simulink model "mdl5"  (R2014a)
settings: Solver=FixedStepDiscrete  SolverMode=SingleTasking  StartTime=TIME(1)  StopTime=TIME(end)  FixedStep=SIMSTEP  RelTol=1e-3
model workspace (MAT data in the model file):
  autoc_mdd_data01 : struct (value not decoded)
values from neighbouring files (symbols this model uses):
  map_mr4_01 = [400 500 600 700 800 900 1000 1100 1200 1300 1400 1500 ... (47 elements, 1x47)]    [scr_simdata_all.mat]
  map_mr4_02 = [0.684 0.622 0.566 0.514 0.468 0.425 0.387 0.352 0.32 0.291 0.264 0.241 ... (47 elements, 1x47)]    [scr_simdata_all.mat]
  map_mr4_03 = [10 12 14 16 18 20 22 24 26 28 30 32 ... (51 elements, 1x51)]    [scr_simdata_all.mat]
  map_mr4_04 = [0.0257 0.0124 0.00595 0.00286 0.00137 0.000662 0.000318 0.000153 7.37e-05 3.54e-05 1.7e-05 8.19e-06 ... (51 elements, 1x51)]    [scr_simdata_all.mat]
  map_mr4_05 = [10 12 14 16 18 20 22 24 26 28 30 32 ... (51 elements, 1x51)]    [scr_simdata_all.mat]
  map_mr4_06 = [0.9647 0.9835 0.9945 0.9994 0.9972 0.9871 0.97 0.9462 0.9163 0.8807 0.8403 0.796 ... (51 elements, 1x51)]    [scr_simdata_all.mat]
  map_mr4_07 = [0 1 2 3 4 5 6 7 8 9 10 11 ... (51 elements, 1x51)]    [scr_simdata_all.mat]
  map_mr4_08 = [0 0.01 0.0214 0.0335 0.0459 0.0587 0.0718 0.085 0.0985 0.112 0.126 0.14 ... (51 elements, 1x51)]    [scr_simdata_all.mat]
  Parameter114 = 126    [scr_simdata_all.mat]
  Parameter115 = 129    [scr_simdata_all.mat]
  Parameter131 = 3    [scr_simdata_all.mat]
  Parameter141 = 0    [scr_simdata_all.mat]
  Parameter143 = 1    [scr_simdata_all.mat]
  Parameter144 = 3    [scr_simdata_all.mat]
  Parameter51 = 0    [scr_simdata_all.mat]
  Parameter52 = 1    [scr_simdata_all.mat]
  Parameter53 = 2    [scr_simdata_all.mat]
  Parameter70 = 30    [scr_simdata_all.mat]
  Parameter71 = 33    [scr_simdata_all.mat]
  Parameter92 = 78    [scr_simdata_all.mat]
  Parameter93 = 81    [scr_simdata_all.mat]
  SIMSTEP = 0.0001024    [scr_simdata_all.mat]
(part 2 of 4)

== system mdl5/SubSystem2611/SubSystem2612/SubSystem2620/SubSystem2621 ==
  note: ***編集禁止***
  element : Inport
  Inside_DSR : DataStoreRead  DataStoreName=DSM320
  Selector : Selector  IndexOptions=Index vector (port)  Indices=[1 3]
  Output : Outport
  wires:
  Selector/1 -> Output/1  "mdl5_SubSystem2611_SubSystem2612_SubSystem2620_SubSystem2621_Selector_1"
  element/1 -> Selector/2
  Inside_DSR/1 -> Selector/1  "mdl5_SubSystem2611_SubSystem2612_SubSystem2620_SubSystem2621_Inside_DSR_1"

== system mdl5/SubSystem2611/SubSystem2612/SubSystem2620/SubSystem2622 ==
  note: ***編集禁止***
  element : Inport
  Inside_DSR : DataStoreRead  DataStoreName=DSM319
  Selector : Selector  IndexOptions=Index vector (port)  Indices=[1 3]
  Output : Outport
  wires:
  Inside_DSR/1 -> Selector/1  "mdl5_SubSystem2611_SubSystem2612_SubSystem2620_SubSystem2622_Inside_DSR_1"
  element/1 -> Selector/2
  Selector/1 -> Output/1  "mdl5_SubSystem2611_SubSystem2612_SubSystem2620_SubSystem2622_Selector_1"

== system mdl5/SubSystem2611/SubSystem2612/SubSystem2620/SubSystem2623 ==
  note: ***編集禁止***
  input : Inport
  element : Inport  Port=2
  Assignment : Assignment  IndexOptions=Index vector (port)  OutputSizes=[1 1]
  Inside_DSR : DataStoreRead  DataStoreName=DSM304
  Inside_DSW : DataStoreWrite  DataStoreName=DSM304
  wires:
  element/1 -> Assignment/3
  input/1 -> Assignment/2
  Inside_DSR/1 -> Assignment/1  "mdl5_SubSystem2611_SubSystem2612_SubSystem2620_SubSystem2623_Inside_DSR_1"
  Assignment/1 -> Inside_DSW/1  "mdl5_SubSystem2611_SubSystem2612_SubSystem2620_SubSystem2623_Assignment_1"

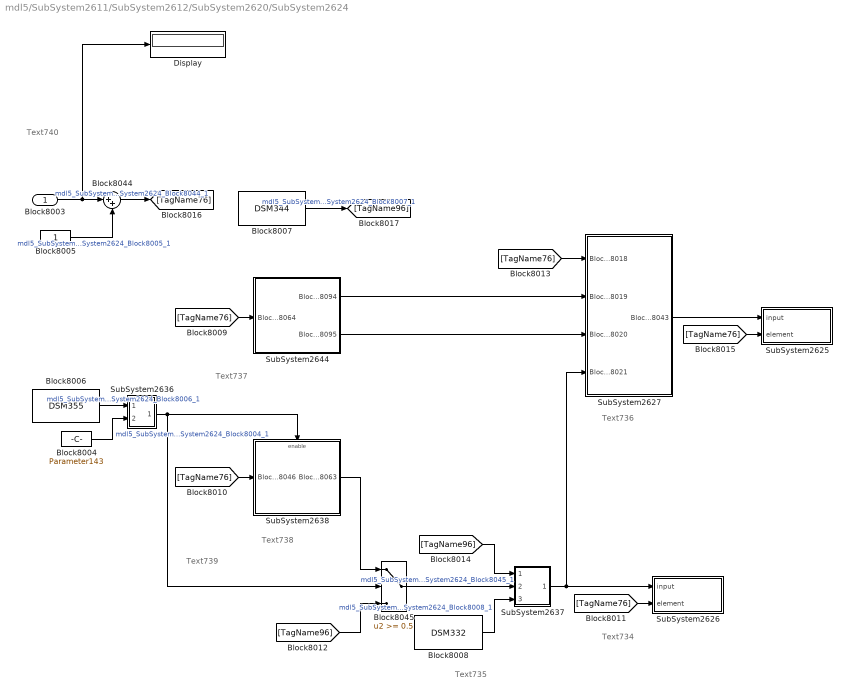
== system mdl5/SubSystem2611/SubSystem2612/SubSystem2620/SubSystem2624 ==
  note: Text740
  note: Text739
  note: Text738
  note: Text737
  note: Text736
  note: Text735
  note: Text734
  Block8003 : Inport
  Block8004 : Constant  Value=Parameter143  OutDataTypeStr=double  SampleTime=-1
  Block8005 : Constant  OutDataTypeStr=double  SampleTime=-1
  Block8006 : DataStoreRead  DataStoreName=DSM355
  Block8007 : DataStoreRead  DataStoreName=DSM344
  Block8008 : DataStoreRead  DataStoreName=DSM332
  Block8044 : Sum  Inputs=|++  OutDataTypeStr=double  RndMeth=Zero  SaturateOnIntegerOverflow=on  InputSameDT=on
  Block8045 : Switch  Threshold=0.5  RndMeth=Zero  SaturateOnIntegerOverflow=on  InputSameDT=on
  Display : Display
  SubSystem2625 : Subsystem  TreatAsAtomicUnit=on  mask(***ATC.DSWVEC***){bd_version=1.01.A, r0=DSM319, r1=-1, r2=, r3=, r4=, r5=, r6=, r7=, r8=, r9=, c0=, c1=, c2=, c3=, c4=, c5=, c6=, c7=, c8=, c9=}
      mask prompts: bd_version "Version"
      mask help: これはAutoCからのブロックです．編集禁止．
      settings: OpenFcn=warndlg('変更禁止!');
      mask Help: web(ui_blockhelpmng(gcb));
      mask Display: disp('ATC.DSRVEC')
  SubSystem2626 : Subsystem  TreatAsAtomicUnit=on  mask(***ATC.DSWVEC***){bd_version=1.01.A, r0=DSM333, r1=-1, r2=, r3=, r4=, r5=, r6=, r7=, r8=, r9=, c0=, c1=, c2=, c3=, c4=, c5=, c6=, c7=, c8=, c9=}
      mask prompts: bd_version "Version"
      mask help: これはAutoCからのブロックです．編集禁止．
      settings: OpenFcn=warndlg('変更禁止!');
      mask Help: web(ui_blockhelpmng(gcb));
      mask Display: disp('ATC.DSRVEC')
  SubSystem2627 : Subsystem  TreatAsAtomicUnit=on
  SubSystem2636 : Subsystem
  SubSystem2637 : Subsystem  TreatAsAtomicUnit=on  mask(***ATC.SATURATION***){bd_version=1.01.A, r0=上下限ガード, r1=上下限ガード, r2=, r3=, r4=, r5=, r6=, r7=, r8=, r9=, c0=, c1=, c2=, c3=, c4=, c5=, c6=, c7=, c8=, c9=}
      mask prompts: bd_version "Version"
      mask help: これはAutoCからのブロックです．編集禁止．
      settings: OpenFcn=warndlg('変更禁止!');  RTWSystemCode=Inline
      mask Help: web(ui_blockhelpmng(gcb));
      mask Display:
      | plot([0 1],[0.5 0.5])
      | plot([0.5 0.5],[0.2 0.8])
      | plot([0.2 0.8],[0.2 0.8])
      | plot([0 0.2],[0.2 0.2])
      | plot([0.8 1],[0.8 0.8])
      | plot([0 0],[0 0])
      | text(0.06,0.9,sprintf('Upper'))
      | plot([0 0],[1 1])
      | text(0.06,0.15,sprintf('Lower'))
  SubSystem2638 : Subsystem  TreatAsAtomicUnit=on
  SubSystem2644 : Subsystem  TreatAsAtomicUnit=on
  wires:
  Block8003/1 -> Display/1, Block8044/1
  Block8006/1 -> SubSystem2636/1(In1)  "mdl5_SubSystem2611_SubSystem2612_SubSystem2620_SubSystem2624_Block8006_1"
  Block8004/1 -> SubSystem2636/2(In2)  "mdl5_SubSystem2611_SubSystem2612_SubSystem2620_SubSystem2624_Block8004_1"
  Block8005/1 -> Block8044/2  "mdl5_SubSystem2611_SubSystem2612_SubSystem2620_SubSystem2624_Block8005_1"
  Block8044/1 -> [TagName76]  "mdl5_SubSystem2611_SubSystem2612_SubSystem2620_SubSystem2624_Block8044_1"
  SubSystem2644/1(Block8094) -> SubSystem2627/2(Block8019)
  SubSystem2644/2(Block8095) -> SubSystem2627/3(Block8020)
  [TagName76] -> SubSystem2627/1(Block8018)
  [TagName76] -> SubSystem2644/1(Block8064)
  [TagName76] -> SubSystem2625/2(element)
  SubSystem2627/1(Block8043) -> SubSystem2625/1(input)
  [TagName76] -> SubSystem2638/1(Block8046)
  SubSystem2636/1(Out1) -> Block8045/2, SubSystem2638/Enable
  [TagName76] -> SubSystem2626/2(element)
  SubSystem2638/1(Block8063) -> Block8045/1
  [TagName96] -> Block8045/3
  Block8045/1 -> SubSystem2637/2(Input)  "mdl5_SubSystem2611_SubSystem2612_SubSystem2620_SubSystem2624_Block8045_1"
  SubSystem2637/1(Output) -> SubSystem2626/1(input), SubSystem2627/4(Block8021)
  Block8008/1 -> SubSystem2637/3(Min)  "mdl5_SubSystem2611_SubSystem2612_SubSystem2620_SubSystem2624_Block8008_1"
  Block8007/1 -> [TagName96]  "mdl5_SubSystem2611_SubSystem2612_SubSystem2620_SubSystem2624_Block8007_1"
  [TagName96] -> SubSystem2637/1(Max)

== system mdl5/SubSystem2611/SubSystem2612/SubSystem2665/SubSystem2666 ==
  note: Text751
  note: Text750
  note: Text749
  note: Text748
  Block8098 : Inport
  Block8099 : Constant  OutDataTypeStr=double  SampleTime=-1
  Block8100 : Constant  Value=2  OutDataTypeStr=double  SampleTime=-1
  Block8101 : Constant  Value=0  OutDataTypeStr=double  SampleTime=-1
  Block8102 : Constant  OutDataTypeStr=double  SampleTime=-1
  Block8103 : DataStoreRead  DataStoreName=DSM327
  Block8108 : Sum  Inputs=++|  OutDataTypeStr=double  RndMeth=Zero  SaturateOnIntegerOverflow=on  InputSameDT=on
  Block8109 : Sum  Inputs=|++  OutDataTypeStr=double  RndMeth=Zero  SaturateOnIntegerOverflow=on  InputSameDT=on
  Block8110 : Switch  Threshold=0.5  RndMeth=Zero  SaturateOnIntegerOverflow=on  InputSameDT=on
  Block8111 : Switch  Threshold=0.5  RndMeth=Zero  SaturateOnIntegerOverflow=on  InputSameDT=on
  SubSystem2667 : Subsystem  TreatAsAtomicUnit=on  mask(***ATC.DSWVEC***){bd_version=1.01.A, r0=DSM320, r1=-1, r2=, r3=, r4=, r5=, r6=, r7=, r8=, r9=, c0=, c1=, c2=, c3=, c4=, c5=, c6=, c7=, c8=, c9=}
      mask prompts: bd_version "Version"
      mask help: これはAutoCからのブロックです．編集禁止．
      settings: OpenFcn=warndlg('変更禁止!');
      mask Help: web(ui_blockhelpmng(gcb));
      mask Display: disp('ATC.DSRVEC')
  SubSystem2668 : Subsystem
  SubSystem2669 : Subsystem
  SubSystem2670 : Subsystem  Priority=1  TreatAsAtomicUnit=on
      settings: AttributesFormatString=Attribute2108
  SubSystem2676 : Subsystem  Priority=10  TreatAsAtomicUnit=on
      settings: AttributesFormatString=Attribute2115
  wires:
  Block8098/1 -> Block8109/1
  SubSystem2669/1(Out1) -> Block8110/2
  Block8103/1 -> SubSystem2669/1(In1), SubSystem2668/1(In1)  "mdl5_SubSystem2611_SubSystem2612_SubSystem2665_SubSystem2666_Block8103_1"
  Block8099/1 -> SubSystem2669/2(In2)  "mdl5_SubSystem2611_SubSystem2612_SubSystem2665_SubSystem2666_Block8099_1"
  Block8100/1 -> SubSystem2668/2(In2)  "mdl5_SubSystem2611_SubSystem2612_SubSystem2665_SubSystem2666_Block8100_1"
  SubSystem2668/1(Out1) -> Block8111/2
  Block8101/1 -> Block8111/3  "mdl5_SubSystem2611_SubSystem2612_SubSystem2665_SubSystem2666_Block8101_1"
  Block8108/1 -> Block8111/1  "mdl5_SubSystem2611_SubSystem2612_SubSystem2665_SubSystem2666_Block8108_1"
  Block8102/1 -> Block8109/2  "mdl5_SubSystem2611_SubSystem2612_SubSystem2665_SubSystem2666_Block8102_1"
  Block8109/1 -> [TagName76]  "mdl5_SubSystem2611_SubSystem2612_SubSystem2665_SubSystem2666_Block8109_1"
  Block8110/1 -> SubSystem2667/1(input)  "mdl5_SubSystem2611_SubSystem2612_SubSystem2665_SubSystem2666_Block8110_1"
  [TagName76] -> SubSystem2667/2(element)
  [TagName76] -> SubSystem2670/1(Block8112)
  Block8111/1 -> Block8110/3  "mdl5_SubSystem2611_SubSystem2612_SubSystem2665_SubSystem2666_Block8111_1"
  SubSystem2670/1(Block8132) -> Block8110/1, Block8108/1
  [TagName76] -> SubSystem2676/1(Block8133)
  SubSystem2676/1(Block8232) -> Block8108/2

== system mdl5/SubSystem2611/SubSystem2691/SubSystem2693/SubSystem2694 ==
  note: ***編集禁止***
  N : Inport
  For_loop : Stateflow chart  TreatAsAtomicUnit=on
  action : Outport
  i : Outport  Port=2
  wires:
  For_loop/1(idx) -> i/1
  N/1 -> For_loop/1(N_Loop)
  For_loop/2(function_call) -> action/1

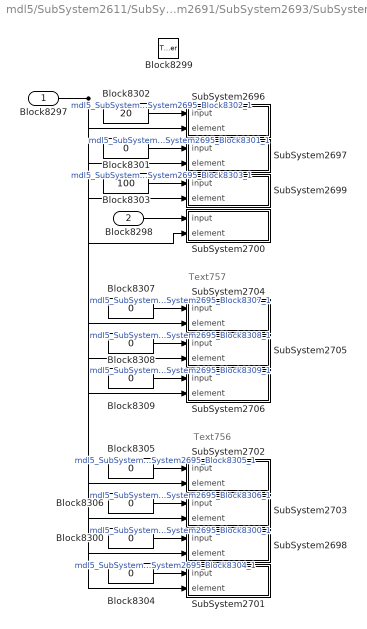
== system mdl5/SubSystem2611/SubSystem2691/SubSystem2693/SubSystem2695 ==
  note: Text757
  note: Text756
  Block8297 : Inport
  Block8298 : Inport  Port=2
  Block8299 : TriggerPort  TriggerType=function-call
  Block{8300..8301,8304..8309} (8 alike) : Constant  Value=0  OutDataTypeStr=double  SampleTime=-1
  Block8302 : Constant  Value=20  OutDataTypeStr=double  SampleTime=-1
  Block8303 : Constant  Value=100  OutDataTypeStr=double  SampleTime=-1
  SubSystem2696 : Subsystem  TreatAsAtomicUnit=on  mask(***ATC.DSWVEC***){bd_version=1.01.A, r0=DSM320, r1=-1, r2=, r3=, r4=, r5=, r6=, r7=, r8=, r9=, c0=, c1=, c2=, c3=, c4=, c5=, c6=, c7=, c8=, c9=}
      mask prompts: bd_version "Version"
      mask help: これはAutoCからのブロックです．編集禁止．
      settings: OpenFcn=warndlg('変更禁止!');
      mask Help: web(ui_blockhelpmng(gcb));
      mask Display: disp('ATC.DSRVEC')
  SubSystem2697 : Subsystem  TreatAsAtomicUnit=on  mask(***ATC.DSWVEC***){bd_version=1.01.A, r0=DSM319, r1=-1, r2=, r3=, r4=, r5=, r6=, r7=, r8=, r9=, c0=, c1=, c2=, c3=, c4=, c5=, c6=, c7=, c8=, c9=}
      mask prompts: bd_version "Version"
      mask help: これはAutoCからのブロックです．編集禁止．
      settings: OpenFcn=warndlg('変更禁止!');
      mask Help: web(ui_blockhelpmng(gcb));
      mask Display: disp('ATC.DSRVEC')
  SubSystem2698 : Subsystem  TreatAsAtomicUnit=on  mask(***ATC.DSWVEC***){bd_version=1.01.A, r0=DSM336, r1=-1, r2=, r3=, r4=, r5=, r6=, r7=, r8=, r9=, c0=, c1=, c2=, c3=, c4=, c5=, c6=, c7=, c8=, c9=}
      mask prompts: bd_version "Version"
      mask help: これはAutoCからのブロックです．編集禁止．
      settings: OpenFcn=warndlg('変更禁止!');
      mask Help: web(ui_blockhelpmng(gcb));
      mask Display: disp('ATC.DSRVEC')
  SubSystem2699 : Subsystem  TreatAsAtomicUnit=on  mask(***ATC.DSWVEC***){bd_version=1.01.A, r0=DSM318, r1=-1, r2=, r3=, r4=, r5=, r6=, r7=, r8=, r9=, c0=, c1=, c2=, c3=, c4=, c5=, c6=, c7=, c8=, c9=}
      mask prompts: bd_version "Version"
      mask help: これはAutoCからのブロックです．編集禁止．
      settings: OpenFcn=warndlg('変更禁止!');
      mask Help: web(ui_blockhelpmng(gcb));
      mask Display: disp('ATC.DSRVEC')
  SubSystem2700 : Subsystem  TreatAsAtomicUnit=on  mask(***ATC.DSWVEC***){bd_version=1.01.A, r0=DSM333, r1=-1, r2=, r3=, r4=, r5=, r6=, r7=, r8=, r9=, c0=, c1=, c2=, c3=, c4=, c5=, c6=, c7=, c8=, c9=}
      mask prompts: bd_version "Version"
      mask help: これはAutoCからのブロックです．編集禁止．
      settings: OpenFcn=warndlg('変更禁止!');
      mask Help: web(ui_blockhelpmng(gcb));
      mask Display: disp('ATC.DSRVEC')
  SubSystem2701 : Subsystem  TreatAsAtomicUnit=on  mask(***ATC.DSWVEC***){bd_version=1.01.A, r0=DSM337, r1=-1, r2=, r3=, r4=, r5=, r6=, r7=, r8=, r9=, c0=, c1=, c2=, c3=, c4=, c5=, c6=, c7=, c8=, c9=}
      mask prompts: bd_version "Version"
      mask help: これはAutoCからのブロックです．編集禁止．
      settings: OpenFcn=warndlg('変更禁止!');
      mask Help: web(ui_blockhelpmng(gcb));
      mask Display: disp('ATC.DSRVEC')
  SubSystem2702 : Subsystem  TreatAsAtomicUnit=on  mask(***ATC.DSWVEC***){bd_version=1.01.A, r0=DSM334, r1=-1, r2=, r3=, r4=, r5=, r6=, r7=, r8=, r9=, c0=, c1=, c2=, c3=, c4=, c5=, c6=, c7=, c8=, c9=}
      mask prompts: bd_version "Version"
      mask help: これはAutoCからのブロックです．編集禁止．
      settings: OpenFcn=warndlg('変更禁止!');
      mask Help: web(ui_blockhelpmng(gcb));
      mask Display: disp('ATC.DSRVEC')
  SubSystem2703 : Subsystem  TreatAsAtomicUnit=on  mask(***ATC.DSWVEC***){bd_version=1.01.A, r0=DSM335, r1=-1, r2=, r3=, r4=, r5=, r6=, r7=, r8=, r9=, c0=, c1=, c2=, c3=, c4=, c5=, c6=, c7=, c8=, c9=}
      mask prompts: bd_version "Version"
      mask help: これはAutoCからのブロックです．編集禁止．
      settings: OpenFcn=warndlg('変更禁止!');
      mask Help: web(ui_blockhelpmng(gcb));
      mask Display: disp('ATC.DSRVEC')
  SubSystem2704 : Subsystem  TreatAsAtomicUnit=on  mask(***ATC.DSWVEC***){bd_version=1.01.A, r0=DSM348, r1=-1, r2=, r3=, r4=, r5=, r6=, r7=, r8=, r9=, c0=, c1=, c2=, c3=, c4=, c5=, c6=, c7=, c8=, c9=}
      mask prompts: bd_version "Version"
      mask help: これはAutoCからのブロックです．編集禁止．
      settings: OpenFcn=warndlg('変更禁止!');
      mask Help: web(ui_blockhelpmng(gcb));
      mask Display: disp('ATC.DSRVEC')
  SubSystem2705 : Subsystem  TreatAsAtomicUnit=on  mask(***ATC.DSWVEC***){bd_version=1.01.A, r0=DSM349, r1=-1, r2=, r3=, r4=, r5=, r6=, r7=, r8=, r9=, c0=, c1=, c2=, c3=, c4=, c5=, c6=, c7=, c8=, c9=}
      mask prompts: bd_version "Version"
      mask help: これはAutoCからのブロックです．編集禁止．
      settings: OpenFcn=warndlg('変更禁止!');
      mask Help: web(ui_blockhelpmng(gcb));
      mask Display: disp('ATC.DSRVEC')
  SubSystem2706 : Subsystem  TreatAsAtomicUnit=on  mask(***ATC.DSWVEC***){bd_version=1.01.A, r0=DSM347, r1=-1, r2=, r3=, r4=, r5=, r6=, r7=, r8=, r9=, c0=, c1=, c2=, c3=, c4=, c5=, c6=, c7=, c8=, c9=}
      mask prompts: bd_version "Version"
      mask help: これはAutoCからのブロックです．編集禁止．
      settings: OpenFcn=warndlg('変更禁止!');
      mask Help: web(ui_blockhelpmng(gcb));
      mask Display: disp('ATC.DSRVEC')
  wires:
  Block8304/1 -> SubSystem2701/1(input)  "mdl5_SubSystem2611_SubSystem2691_SubSystem2693_SubSystem2695_Block8304_1"
  Block8305/1 -> SubSystem2702/1(input)  "mdl5_SubSystem2611_SubSystem2691_SubSystem2693_SubSystem2695_Block8305_1"
  Block8306/1 -> SubSystem2703/1(input)  "mdl5_SubSystem2611_SubSystem2691_SubSystem2693_SubSystem2695_Block8306_1"
  Block8300/1 -> SubSystem2698/1(input)  "mdl5_SubSystem2611_SubSystem2691_SubSystem2693_SubSystem2695_Block8300_1"
  Block8298/1 -> SubSystem2700/1(input)
  Block8302/1 -> SubSystem2696/1(input)  "mdl5_SubSystem2611_SubSystem2691_SubSystem2693_SubSystem2695_Block8302_1"
  Block8297/1 -> SubSystem2701/2(element), SubSystem2698/2(element), SubSystem2703/2(element), SubSystem2702/2(element), SubSystem2700/2(element), SubSystem2696/2(element), SubSystem2699/2(element), SubSystem2697/2(element), SubSystem2704/2(element), SubSystem2705/2(element), SubSystem2706/2(element)
  Block8301/1 -> SubSystem2697/1(input)  "mdl5_SubSystem2611_SubSystem2691_SubSystem2693_SubSystem2695_Block8301_1"
  Block8303/1 -> SubSystem2699/1(input)  "mdl5_SubSystem2611_SubSystem2691_SubSystem2693_SubSystem2695_Block8303_1"
  Block8307/1 -> SubSystem2704/1(input)  "mdl5_SubSystem2611_SubSystem2691_SubSystem2693_SubSystem2695_Block8307_1"
  Block8308/1 -> SubSystem2705/1(input)  "mdl5_SubSystem2611_SubSystem2691_SubSystem2693_SubSystem2695_Block8308_1"
  Block8309/1 -> SubSystem2706/1(input)  "mdl5_SubSystem2611_SubSystem2691_SubSystem2693_SubSystem2695_Block8309_1"

== system mdl5/SubSystem2611/SubSystem2612/SubSystem2620/SubSystem2624/SubSystem2625 ==
  note: ***編集禁止***
  input : Inport
  element : Inport  Port=2
  Assignment : Assignment  IndexOptions=Index vector (port)  OutputSizes=[1 1]
  Inside_DSR : DataStoreRead  DataStoreName=DSM319
  Inside_DSW : DataStoreWrite  DataStoreName=DSM319
  wires:
  element/1 -> Assignment/3
  input/1 -> Assignment/2
  Inside_DSR/1 -> Assignment/1  "mdl5_SubSystem2611_SubSystem2612_SubSystem2620_SubSystem2624_SubSystem2625_Inside_DSR_1"
  Assignment/1 -> Inside_DSW/1  "mdl5_SubSystem2611_SubSystem2612_SubSystem2620_SubSystem2624_SubSystem2625_Assignment_1"

== system mdl5/SubSystem2611/SubSystem2612/SubSystem2620/SubSystem2624/SubSystem2626 ==
  note: ***編集禁止***
  input : Inport
  element : Inport  Port=2
  Assignment : Assignment  IndexOptions=Index vector (port)  OutputSizes=[1 1]
  Inside_DSR : DataStoreRead  DataStoreName=DSM333
  Inside_DSW : DataStoreWrite  DataStoreName=DSM333
  wires:
  element/1 -> Assignment/3
  input/1 -> Assignment/2
  Inside_DSR/1 -> Assignment/1  "mdl5_SubSystem2611_SubSystem2612_SubSystem2620_SubSystem2624_SubSystem2626_Inside_DSR_1"
  Assignment/1 -> Inside_DSW/1  "mdl5_SubSystem2611_SubSystem2612_SubSystem2620_SubSystem2624_SubSystem2626_Assignment_1"

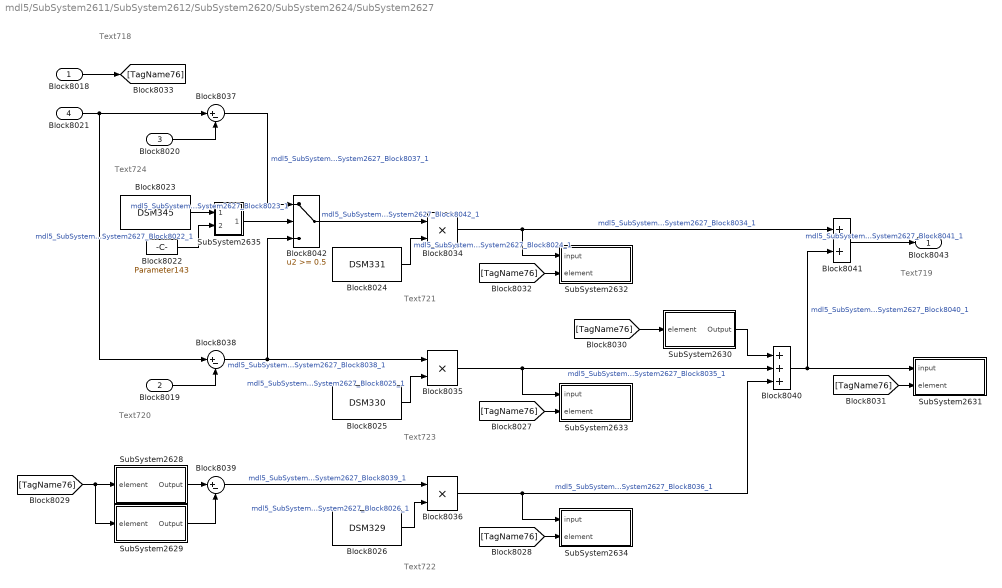
== system mdl5/SubSystem2611/SubSystem2612/SubSystem2620/SubSystem2624/SubSystem2627 ==
  note: Text724
  note: Text723
  note: Text722
  note: Text721
  note: Text720
  note: Text719
  note: Text718
  Block8018 : Inport
  Block8019 : Inport  Port=2
  Block8020 : Inport  Port=3
  Block8021 : Inport  Port=4
  Block8022 : Constant  Value=Parameter143  OutDataTypeStr=double  SampleTime=-1
  Block8023 : DataStoreRead  DataStoreName=DSM345
  Block8024 : DataStoreRead  DataStoreName=DSM331
  Block8025 : DataStoreRead  DataStoreName=DSM330
  Block8026 : DataStoreRead  DataStoreName=DSM329
  Block8034 : Product  OutDataTypeStr=double  SaturateOnIntegerOverflow=on  RndMeth=Zero  InputSameDT=on
  Block8035 : Product  OutDataTypeStr=double  SaturateOnIntegerOverflow=on  RndMeth=Zero  InputSameDT=on
  Block8036 : Product  OutDataTypeStr=double  SaturateOnIntegerOverflow=on  RndMeth=Zero  InputSameDT=on
  Block8037 : Sum  Inputs=|+-  OutDataTypeStr=double  RndMeth=Zero  SaturateOnIntegerOverflow=on  InputSameDT=on
  Block8038 : Sum  Inputs=|+-  OutDataTypeStr=double  RndMeth=Zero  SaturateOnIntegerOverflow=on  InputSameDT=on
  Block8039 : Sum  Inputs=|+-  OutDataTypeStr=double  RndMeth=Zero  SaturateOnIntegerOverflow=on  InputSameDT=on
  Block8040 : Sum  Inputs=+++  OutDataTypeStr=double  RndMeth=Zero  SaturateOnIntegerOverflow=on  InputSameDT=on
  Block8041 : Sum  OutDataTypeStr=double  RndMeth=Zero  SaturateOnIntegerOverflow=on  InputSameDT=on
  Block8042 : Switch  Threshold=0.5  RndMeth=Zero  SaturateOnIntegerOverflow=on  InputSameDT=on
  SubSystem2628 : Subsystem  TreatAsAtomicUnit=on  mask(***ATC.DSRVEC***){bd_version=1.01.A, r0=DSM147, r1=-1, r2=, r3=, r4=, r5=, r6=, r7=, r8=, r9=, c0=, c1=, c2=, c3=, c4=, c5=, c6=, c7=, c8=, c9=}
      mask prompts: bd_version "Version"
      mask help: これはAutoCからのブロックです．編集禁止．
      settings: OpenFcn=warndlg('変更禁止!');
      mask Help: web(ui_blockhelpmng(gcb));
      mask Display: disp('ATC.DSRVEC')
  SubSystem2629 : Subsystem  TreatAsAtomicUnit=on  mask(***ATC.DSRVEC***){bd_version=1.01.A, r0=DSM304, r1=-1, r2=, r3=, r4=, r5=, r6=, r7=, r8=, r9=, c0=, c1=, c2=, c3=, c4=, c5=, c6=, c7=, c8=, c9=}
      mask prompts: bd_version "Version"
      mask help: これはAutoCからのブロックです．編集禁止．
      settings: OpenFcn=warndlg('変更禁止!');
      mask Help: web(ui_blockhelpmng(gcb));
      mask Display: disp('ATC.DSRVEC')
  SubSystem2630 : Subsystem  Priority=1  TreatAsAtomicUnit=on  mask(***ATC.DSRVEC***){bd_version=1.01.A, r0=DSM346, r1=-1, r2=, r3=, r4=, r5=, r6=, r7=, r8=, r9=, c0=, c1=, c2=, c3=, c4=, c5=, c6=, c7=, c8=, c9=}
      mask prompts: bd_version "Version"
      mask help: これはAutoCからのブロックです．編集禁止．
      settings: AttributesFormatString=Attribute2091  OpenFcn=warndlg('変更禁止!');
      mask Help: web(ui_blockhelpmng(gcb));
      mask Display: disp('ATC.DSRVEC')
  SubSystem2631 : Subsystem  Priority=10  TreatAsAtomicUnit=on  mask(***ATC.DSWVEC***){bd_version=1.01.A, r0=DSM346, r1=-1, r2=, r3=, r4=, r5=, r6=, r7=, r8=, r9=, c0=, c1=, c2=, c3=, c4=, c5=, c6=, c7=, c8=, c9=}
      mask prompts: bd_version "Version"
      mask help: これはAutoCからのブロックです．編集禁止．
      settings: AttributesFormatString=Attribute2092  OpenFcn=warndlg('変更禁止!');
      mask Help: web(ui_blockhelpmng(gcb));
      mask Display: disp('ATC.DSRVEC')
  SubSystem2632 : Subsystem  TreatAsAtomicUnit=on  mask(***ATC.DSWVEC***){bd_version=1.01.A, r0=DSM349, r1=-1, r2=, r3=, r4=, r5=, r6=, r7=, r8=, r9=, c0=, c1=, c2=, c3=, c4=, c5=, c6=, c7=, c8=, c9=}
      mask prompts: bd_version "Version"
      mask help: これはAutoCからのブロックです．編集禁止．
      settings: OpenFcn=warndlg('変更禁止!');
      mask Help: web(ui_blockhelpmng(gcb));
      mask Display: disp('ATC.DSRVEC')
  SubSystem2633 : Subsystem  TreatAsAtomicUnit=on  mask(***ATC.DSWVEC***){bd_version=1.01.A, r0=DSM348, r1=-1, r2=, r3=, r4=, r5=, r6=, r7=, r8=, r9=, c0=, c1=, c2=, c3=, c4=, c5=, c6=, c7=, c8=, c9=}
      mask prompts: bd_version "Version"
      mask help: これはAutoCからのブロックです．編集禁止．
      settings: OpenFcn=warndlg('変更禁止!');
      mask Help: web(ui_blockhelpmng(gcb));
      mask Display: disp('ATC.DSRVEC')
  SubSystem2634 : Subsystem  TreatAsAtomicUnit=on  mask(***ATC.DSWVEC***){bd_version=1.01.A, r0=DSM347, r1=-1, r2=, r3=, r4=, r5=, r6=, r7=, r8=, r9=, c0=, c1=, c2=, c3=, c4=, c5=, c6=, c7=, c8=, c9=}
      mask prompts: bd_version "Version"
      mask help: これはAutoCからのブロックです．編集禁止．
      settings: OpenFcn=warndlg('変更禁止!');
      mask Help: web(ui_blockhelpmng(gcb));
      mask Display: disp('ATC.DSRVEC')
  SubSystem2635 : Subsystem
  Block8043 : Outport
  wires:
  [TagName76] -> SubSystem2629/1(element), SubSystem2628/1(element)
  SubSystem2629/1(Output) -> Block8039/2
  SubSystem2628/1(Output) -> Block8039/1
  Block8023/1 -> SubSystem2635/1(In1)  "mdl5_SubSystem2611_SubSystem2612_SubSystem2620_SubSystem2624_SubSystem2627_Block8023_1"
  Block8022/1 -> SubSystem2635/2(In2)  "mdl5_SubSystem2611_SubSystem2612_SubSystem2620_SubSystem2624_SubSystem2627_Block8022_1"
  Block8019/1 -> Block8038/2
  Block8020/1 -> Block8037/2
  Block8021/1 -> Block8037/1, Block8038/1
  SubSystem2635/1(Out1) -> Block8042/2
  Block8037/1 -> Block8042/1  "mdl5_SubSystem2611_SubSystem2612_SubSystem2620_SubSystem2624_SubSystem2627_Block8037_1"
  Block8038/1 -> Block8042/3, Block8035/1  "mdl5_SubSystem2611_SubSystem2612_SubSystem2620_SubSystem2624_SubSystem2627_Block8038_1"
  Block8042/1 -> Block8034/1  "mdl5_SubSystem2611_SubSystem2612_SubSystem2620_SubSystem2624_SubSystem2627_Block8042_1"
  Block8024/1 -> Block8034/2  "mdl5_SubSystem2611_SubSystem2612_SubSystem2620_SubSystem2624_SubSystem2627_Block8024_1"
  Block8025/1 -> Block8035/2  "mdl5_SubSystem2611_SubSystem2612_SubSystem2620_SubSystem2624_SubSystem2627_Block8025_1"
  Block8026/1 -> Block8036/2  "mdl5_SubSystem2611_SubSystem2612_SubSystem2620_SubSystem2624_SubSystem2627_Block8026_1"
  Block8039/1 -> Block8036/1  "mdl5_SubSystem2611_SubSystem2612_SubSystem2620_SubSystem2624_SubSystem2627_Block8039_1"
  Block8036/1 -> Block8040/3, SubSystem2634/1(input)  "mdl5_SubSystem2611_SubSystem2612_SubSystem2620_SubSystem2624_SubSystem2627_Block8036_1"
  Block8034/1 -> Block8041/1, SubSystem2632/1(input)  "mdl5_SubSystem2611_SubSystem2612_SubSystem2620_SubSystem2624_SubSystem2627_Block8034_1"
  Block8040/1 -> Block8041/2, SubSystem2631/1(input)  "mdl5_SubSystem2611_SubSystem2612_SubSystem2620_SubSystem2624_SubSystem2627_Block8040_1"
  [TagName76] -> SubSystem2630/1(element)
  Block8035/1 -> Block8040/2, SubSystem2633/1(input)  "mdl5_SubSystem2611_SubSystem2612_SubSystem2620_SubSystem2624_SubSystem2627_Block8035_1"
  SubSystem2630/1(Output) -> Block8040/1
  Block8041/1 -> Block8043/1  "mdl5_SubSystem2611_SubSystem2612_SubSystem2620_SubSystem2624_SubSystem2627_Block8041_1"
  [TagName76] -> SubSystem2631/2(element)
  [TagName76] -> SubSystem2632/2(element)
  [TagName76] -> SubSystem2633/2(element)
  [TagName76] -> SubSystem2634/2(element)
  Block8018/1 -> [TagName76]

== system mdl5/SubSystem2611/SubSystem2612/SubSystem2620/SubSystem2624/SubSystem2636 ==
  note: ***編集禁止***
  In1 : Inport
  In2 : Inport  Port=2
  RO1 : RelationalOperator  Operator===  InputSameDT=on
  single1 : DataTypeConversion  OutDataTypeStr=single  SaturateOnIntegerOverflow=on  RndMeth=Zero
  single2 : DataTypeConversion  OutDataTypeStr=single  SaturateOnIntegerOverflow=on  RndMeth=Zero
  Out1 : Outport
  wires:
  RO1/1 -> Out1/1  "mdl5_SubSystem2611_SubSystem2612_SubSystem2620_SubSystem2624_SubSystem2636_RO1_1"
  In2/1 -> single2/1
  In1/1 -> single1/1
  single1/1 -> RO1/1  "mdl5_SubSystem2611_SubSystem2612_SubSystem2620_SubSystem2624_SubSystem2636_single1_1"
  single2/1 -> RO1/2  "mdl5_SubSystem2611_SubSystem2612_SubSystem2620_SubSystem2624_SubSystem2636_single2_1"

== system mdl5/SubSystem2611/SubSystem2612/SubSystem2620/SubSystem2624/SubSystem2637 ==
  note: ***編集禁止***
  Max : Inport
  Input : Inport  Port=2
  Min : Inport  Port=3
  Max1 : MinMax  Function=max  Inputs=2  SaturateOnIntegerOverflow=on  InputSameDT=on
  Min1 : MinMax  Inputs=2  SaturateOnIntegerOverflow=on  InputSameDT=on
  Output : Outport
  wires:
  Min1/1 -> Output/1  "mdl5_SubSystem2611_SubSystem2612_SubSystem2620_SubSystem2624_SubSystem2637_Min1_1"
  Max/1 -> Min1/1
  Input/1 -> Max1/1
  Min/1 -> Max1/2
  Max1/1 -> Min1/2  "mdl5_SubSystem2611_SubSystem2612_SubSystem2620_SubSystem2624_SubSystem2637_Max1_1"

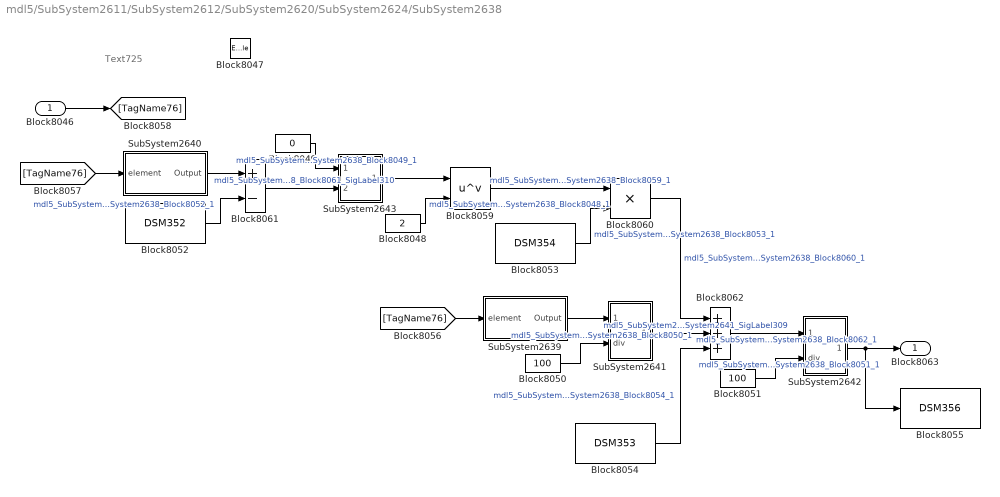
== system mdl5/SubSystem2611/SubSystem2612/SubSystem2620/SubSystem2624/SubSystem2638 ==
  note: Text725
  Block8046 : Inport
  Block8047 : EnablePort
  Block8048 : Constant  Value=2  OutDataTypeStr=double  SampleTime=-1
  Block8049 : Constant  Value=0  OutDataTypeStr=double  SampleTime=-1
  Block8050 : Constant  Value=100  OutDataTypeStr=double  SampleTime=-1
  Block8051 : Constant  Value=100  OutDataTypeStr=double  SampleTime=-1
  Block8052 : DataStoreRead  DataStoreName=DSM352
  Block8053 : DataStoreRead  DataStoreName=DSM354
  Block8054 : DataStoreRead  DataStoreName=DSM353
  Block8055 : DataStoreWrite  DataStoreName=DSM356
  Block8059 : Math  Operator=pow  SaturateOnIntegerOverflow=on
  Block8060 : Product  OutDataTypeStr=double  SaturateOnIntegerOverflow=on  RndMeth=Zero  InputSameDT=on
  Block8061 : Sum  Inputs=+-  OutDataTypeStr=double  RndMeth=Zero  SaturateOnIntegerOverflow=on  InputSameDT=on
  Block8062 : Sum  Inputs=+++  OutDataTypeStr=double  RndMeth=Zero  SaturateOnIntegerOverflow=on  InputSameDT=on
  SubSystem2639 : Subsystem  TreatAsAtomicUnit=on  mask(***ATC.DSRVEC***){bd_version=1.01.A, r0=DSM97, r1=-1, r2=, r3=, r4=, r5=, r6=, r7=, r8=, r9=, c0=, c1=, c2=, c3=, c4=, c5=, c6=, c7=, c8=, c9=}
      mask prompts: bd_version "Version"
      mask help: これはAutoCからのブロックです．編集禁止．
      settings: OpenFcn=warndlg('変更禁止!');
      mask Help: web(ui_blockhelpmng(gcb));
      mask Display: disp('ATC.DSRVEC')
  SubSystem2640 : Subsystem  TreatAsAtomicUnit=on  mask(***ATC.DSRVEC***){bd_version=1.01.A, r0=DSM318, r1=-1, r2=, r3=, r4=, r5=, r6=, r7=, r8=, r9=, c0=, c1=, c2=, c3=, c4=, c5=, c6=, c7=, c8=, c9=}
      mask prompts: bd_version "Version"
      mask help: これはAutoCからのブロックです．編集禁止．
      settings: OpenFcn=warndlg('変更禁止!');
      mask Help: web(ui_blockhelpmng(gcb));
      mask Display: disp('ATC.DSRVEC')
  SubSystem2641 : Subsystem  TreatAsAtomicUnit=on  mask(***ATC.DIVISION***){bd_version=1.01.A, r0=チェック無し, r1=, r2=, r3=, r4=, r5=, r6=, r7=, r8=, r9=, c0=, c1=, c2=, c3=, c4=, c5=, c6=, c7=, c8=, c9=}
      mask prompts: bd_version "Version"
      mask help: これはAutoCからのブロックです．編集禁止．
      settings: OpenFcn=warndlg('変更禁止!');
      mask Help: web(ui_blockhelpmng(gcb));
  SubSystem2642 : Subsystem  TreatAsAtomicUnit=on  mask(***ATC.DIVISION***){bd_version=1.01.A, r0=チェック無し, r1=, r2=, r3=, r4=, r5=, r6=, r7=, r8=, r9=, c0=, c1=, c2=, c3=, c4=, c5=, c6=, c7=, c8=, c9=}
      mask prompts: bd_version "Version"
      mask help: これはAutoCからのブロックです．編集禁止．
      settings: OpenFcn=warndlg('変更禁止!');
      mask Help: web(ui_blockhelpmng(gcb));
  SubSystem2643 : Subsystem  TreatAsAtomicUnit=on  mask(***ATC.SATURATION***){bd_version=1.01.A, r0=上限ガード, r1=上限ガード, r2=, r3=, r4=, r5=, r6=, r7=, r8=, r9=, c0=, c1=, c2=, c3=, c4=, c5=, c6=, c7=, c8=, c9=}
      mask prompts: bd_version "Version"
      mask help: これはAutoCからのブロックです．編集禁止．
      settings: OpenFcn=warndlg('変更禁止!');  RTWSystemCode=Inline
      mask Help: web(ui_blockhelpmng(gcb));
      mask Display:
      | plot([0 1],[0.3 0.3])
      | plot([0.5 0.5],[0 0.8])
      | plot([0.2 0.8],[0 0.7])
      | plot([0.8 1],[0.7 0.7])
      | plot([0 0],[1 1])
      | text(0.06,0.9,sprintf('Upper'))
  Block8063 : Outport
  wires:
  [TagName76] -> SubSystem2640/1(element)
  SubSystem2640/1(Output) -> Block8061/1
  Block8061/1 -> SubSystem2643/2(Input)  "mdl5_SubSystem2611_SubSystem2612_SubSystem2620_SubSystem2624_SubSystem2638_Block8061_SigLabel310"
  Block8049/1 -> SubSystem2643/1(Max)  "mdl5_SubSystem2611_SubSystem2612_SubSystem2620_SubSystem2624_SubSystem2638_Block8049_1"
  Block8053/1 -> Block8060/2  "mdl5_SubSystem2611_SubSystem2612_SubSystem2620_SubSystem2624_SubSystem2638_Block8053_1"
  Block8052/1 -> Block8061/2  "mdl5_SubSystem2611_SubSystem2612_SubSystem2620_SubSystem2624_SubSystem2638_Block8052_1"
  Block8054/1 -> Block8062/3  "mdl5_SubSystem2611_SubSystem2612_SubSystem2620_SubSystem2624_SubSystem2638_Block8054_1"
  Block8046/1 -> [TagName76]
  Block8059/1 -> Block8060/1  "mdl5_SubSystem2611_SubSystem2612_SubSystem2620_SubSystem2624_SubSystem2638_Block8059_1"
  SubSystem2643/1(Output) -> Block8059/1
  Block8048/1 -> Block8059/2  "mdl5_SubSystem2611_SubSystem2612_SubSystem2620_SubSystem2624_SubSystem2638_Block8048_1"
  SubSystem2639/1(Output) -> SubSystem2641/1(mult)
  Block8050/1 -> SubSystem2641/2(div)  "mdl5_SubSystem2611_SubSystem2612_SubSystem2620_SubSystem2624_SubSystem2638_Block8050_1"
  Block8060/1 -> Block8062/1  "mdl5_SubSystem2611_SubSystem2612_SubSystem2620_SubSystem2624_SubSystem2638_Block8060_1"
  SubSystem2641/1(Out) -> Block8062/2  "mdl5_SubSystem2611_SubSystem2612_SubSystem2620_SubSystem2624_SubSystem2638_SubSystem2641_SigLabel309"
  [TagName76] -> SubSystem2639/1(element)
  Block8051/1 -> SubSystem2642/2(div)  "mdl5_SubSystem2611_SubSystem2612_SubSystem2620_SubSystem2624_SubSystem2638_Block8051_1"
  Block8062/1 -> SubSystem2642/1(mult)  "mdl5_SubSystem2611_SubSystem2612_SubSystem2620_SubSystem2624_SubSystem2638_Block8062_1"
  SubSystem2642/1(Out) -> Block8063/1, Block8055/1

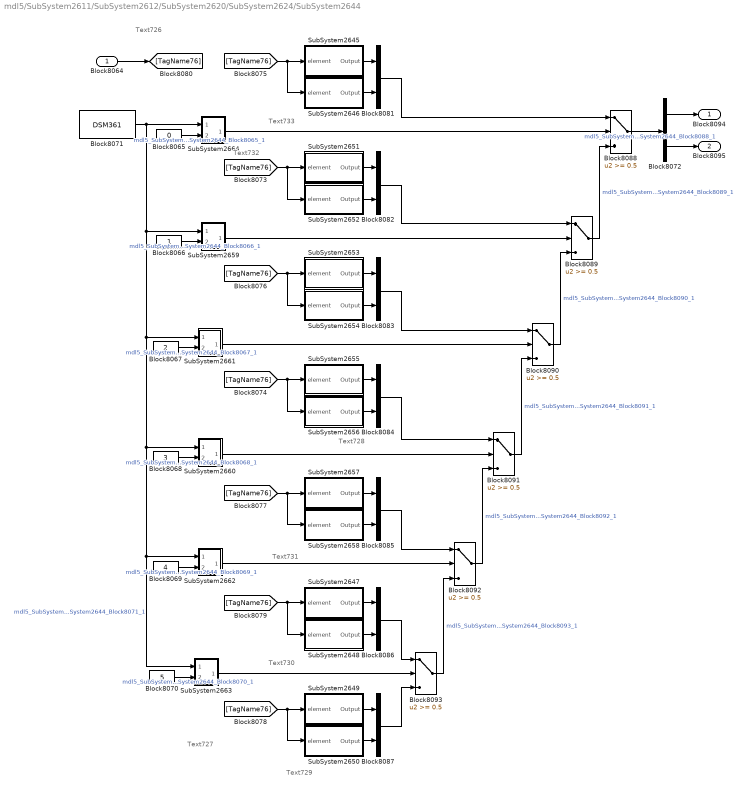
== system mdl5/SubSystem2611/SubSystem2612/SubSystem2620/SubSystem2624/SubSystem2644 ==
  note: Text733
  note: Text732
  note: Text731
  note: Text730
  note: Text729
  note: Text728
  note: Text727
  note: Text726
  Block8064 : Inport
  Block8065 : Constant  Value=0  OutDataTypeStr=double  SampleTime=-1
  Block8066 : Constant  OutDataTypeStr=double  SampleTime=-1
  Block8067 : Constant  Value=2  OutDataTypeStr=double  SampleTime=-1
  Block8068 : Constant  Value=3  OutDataTypeStr=double  SampleTime=-1
  Block8069 : Constant  Value=4  OutDataTypeStr=double  SampleTime=-1
  Block8070 : Constant  Value=5  OutDataTypeStr=double  SampleTime=-1
  Block8071 : DataStoreRead  DataStoreName=DSM361
  Block8072 : Demux  Outputs=2
  Block{8081..8087} (7 alike) : Mux  Inputs=2
  Block{8088..8093} (6 alike) : Switch  Threshold=0.5  RndMeth=Zero  SaturateOnIntegerOverflow=on  InputSameDT=on
  SubSystem2645 : Subsystem  TreatAsAtomicUnit=on  mask(***ATC.DSRVEC***){bd_version=1.01.A, r0=DSM115, r1=-1, r2=, r3=, r4=, r5=, r6=, r7=, r8=, r9=, c0=, c1=, c2=, c3=, c4=, c5=, c6=, c7=, c8=, c9=}
      mask prompts: bd_version "Version"
      mask help: これはAutoCからのブロックです．編集禁止．
      settings: OpenFcn=warndlg('変更禁止!');
      mask Help: web(ui_blockhelpmng(gcb));
      mask Display: disp('ATC.DSRVEC')
  SubSystem2646 : Subsystem  TreatAsAtomicUnit=on  mask(***ATC.DSRVEC***){bd_version=1.01.A, r0=DSM119, r1=-1, r2=, r3=, r4=, r5=, r6=, r7=, r8=, r9=, c0=, c1=, c2=, c3=, c4=, c5=, c6=, c7=, c8=, c9=}
      mask prompts: bd_version "Version"
      mask help: これはAutoCからのブロックです．編集禁止．
      settings: OpenFcn=warndlg('変更禁止!');
      mask Help: web(ui_blockhelpmng(gcb));
      mask Display: disp('ATC.DSRVEC')
  SubSystem2647 : Subsystem  TreatAsAtomicUnit=on  mask(***ATC.DSRVEC***){bd_version=1.01.A, r0=DSM102, r1=-1, r2=, r3=, r4=, r5=, r6=, r7=, r8=, r9=, c0=, c1=, c2=, c3=, c4=, c5=, c6=, c7=, c8=, c9=}
      mask prompts: bd_version "Version"
      mask help: これはAutoCからのブロックです．編集禁止．
      settings: OpenFcn=warndlg('変更禁止!');
      mask Help: web(ui_blockhelpmng(gcb));
      mask Display: disp('ATC.DSRVEC')
  SubSystem2648 : Subsystem  TreatAsAtomicUnit=on  mask(***ATC.DSRVEC***){bd_version=1.01.A, r0=DSM104, r1=-1, r2=, r3=, r4=, r5=, r6=, r7=, r8=, r9=, c0=, c1=, c2=, c3=, c4=, c5=, c6=, c7=, c8=, c9=}
      mask prompts: bd_version "Version"
      mask help: これはAutoCからのブロックです．編集禁止．
      settings: OpenFcn=warndlg('変更禁止!');
      mask Help: web(ui_blockhelpmng(gcb));
      mask Display: disp('ATC.DSRVEC')
  SubSystem2649 : Subsystem  TreatAsAtomicUnit=on  mask(***ATC.DSRVEC***){bd_version=1.01.A, r0=DSM110, r1=-1, r2=, r3=, r4=, r5=, r6=, r7=, r8=, r9=, c0=, c1=, c2=, c3=, c4=, c5=, c6=, c7=, c8=, c9=}
      mask prompts: bd_version "Version"
      mask help: これはAutoCからのブロックです．編集禁止．
      settings: OpenFcn=warndlg('変更禁止!');
      mask Help: web(ui_blockhelpmng(gcb));
      mask Display: disp('ATC.DSRVEC')
  SubSystem2650 : Subsystem  TreatAsAtomicUnit=on  mask(***ATC.DSRVEC***){bd_version=1.01.A, r0=DSM112, r1=-1, r2=, r3=, r4=, r5=, r6=, r7=, r8=, r9=, c0=, c1=, c2=, c3=, c4=, c5=, c6=, c7=, c8=, c9=}
      mask prompts: bd_version "Version"
      mask help: これはAutoCからのブロックです．編集禁止．
      settings: OpenFcn=warndlg('変更禁止!');
      mask Help: web(ui_blockhelpmng(gcb));
      mask Display: disp('ATC.DSRVEC')
  SubSystem2651 : Subsystem  TreatAsAtomicUnit=on  mask(***ATC.DSRVEC***){bd_version=1.01.A, r0=DSM116, r1=-1, r2=, r3=, r4=, r5=, r6=, r7=, r8=, r9=, c0=, c1=, c2=, c3=, c4=, c5=, c6=, c7=, c8=, c9=}
      mask prompts: bd_version "Version"
      mask help: これはAutoCからのブロックです．編集禁止．
      settings: OpenFcn=warndlg('変更禁止!');
      mask Help: web(ui_blockhelpmng(gcb));
      mask Display: disp('ATC.DSRVEC')
  SubSystem2652 : Subsystem  TreatAsAtomicUnit=on  mask(***ATC.DSRVEC***){bd_version=1.01.A, r0=DSM120, r1=-1, r2=, r3=, r4=, r5=, r6=, r7=, r8=, r9=, c0=, c1=, c2=, c3=, c4=, c5=, c6=, c7=, c8=, c9=}
      mask prompts: bd_version "Version"
      mask help: これはAutoCからのブロックです．編集禁止．
      settings: OpenFcn=warndlg('変更禁止!');
      mask Help: web(ui_blockhelpmng(gcb));
      mask Display: disp('ATC.DSRVEC')
  SubSystem2653 : Subsystem  TreatAsAtomicUnit=on  mask(***ATC.DSRVEC***){bd_version=1.01.A, r0=DSM122, r1=-1, r2=, r3=, r4=, r5=, r6=, r7=, r8=, r9=, c0=, c1=, c2=, c3=, c4=, c5=, c6=, c7=, c8=, c9=}
      mask prompts: bd_version "Version"
      mask help: これはAutoCからのブロックです．編集禁止．
      settings: OpenFcn=warndlg('変更禁止!');
      mask Help: web(ui_blockhelpmng(gcb));
      mask Display: disp('ATC.DSRVEC')
  SubSystem2654 : Subsystem  TreatAsAtomicUnit=on  mask(***ATC.DSRVEC***){bd_version=1.01.A, r0=DSM125, r1=-1, r2=, r3=, r4=, r5=, r6=, r7=, r8=, r9=, c0=, c1=, c2=, c3=, c4=, c5=, c6=, c7=, c8=, c9=}
      mask prompts: bd_version "Version"
      mask help: これはAutoCからのブロックです．編集禁止．
      settings: OpenFcn=warndlg('変更禁止!');
      mask Help: web(ui_blockhelpmng(gcb));
      mask Display: disp('ATC.DSRVEC')
  SubSystem2655 : Subsystem  TreatAsAtomicUnit=on  mask(***ATC.DSRVEC***){bd_version=1.01.A, r0=DSM123, r1=-1, r2=, r3=, r4=, r5=, r6=, r7=, r8=, r9=, c0=, c1=, c2=, c3=, c4=, c5=, c6=, c7=, c8=, c9=}
      mask prompts: bd_version "Version"
      mask help: これはAutoCからのブロックです．編集禁止．
      settings: OpenFcn=warndlg('変更禁止!');
      mask Help: web(ui_blockhelpmng(gcb));
      mask Display: disp('ATC.DSRVEC')
  SubSystem2656 : Subsystem  TreatAsAtomicUnit=on  mask(***ATC.DSRVEC***){bd_version=1.01.A, r0=DSM126, r1=-1, r2=, r3=, r4=, r5=, r6=, r7=, r8=, r9=, c0=, c1=, c2=, c3=, c4=, c5=, c6=, c7=, c8=, c9=}
      mask prompts: bd_version "Version"
      mask help: これはAutoCからのブロックです．編集禁止．
      settings: OpenFcn=warndlg('変更禁止!');
      mask Help: web(ui_blockhelpmng(gcb));
      mask Display: disp('ATC.DSRVEC')
  SubSystem2657 : Subsystem  TreatAsAtomicUnit=on  mask(***ATC.DSRVEC***){bd_version=1.01.A, r0=DSM106, r1=-1, r2=, r3=, r4=, r5=, r6=, r7=, r8=, r9=, c0=, c1=, c2=, c3=, c4=, c5=, c6=, c7=, c8=, c9=}
      mask prompts: bd_version "Version"
      mask help: これはAutoCからのブロックです．編集禁止．
      settings: OpenFcn=warndlg('変更禁止!');
      mask Help: web(ui_blockhelpmng(gcb));
      mask Display: disp('ATC.DSRVEC')
  SubSystem2658 : Subsystem  TreatAsAtomicUnit=on  mask(***ATC.DSRVEC***){bd_version=1.01.A, r0=DSM108, r1=-1, r2=, r3=, r4=, r5=, r6=, r7=, r8=, r9=, c0=, c1=, c2=, c3=, c4=, c5=, c6=, c7=, c8=, c9=}
      mask prompts: bd_version "Version"
      mask help: これはAutoCからのブロックです．編集禁止．
      settings: OpenFcn=warndlg('変更禁止!');
      mask Help: web(ui_blockhelpmng(gcb));
      mask Display: disp('ATC.DSRVEC')
  SubSystem2659 : Subsystem
  SubSystem2660 : Subsystem
  SubSystem2661 : Subsystem
  SubSystem2662 : Subsystem
  SubSystem2663 : Subsystem
  SubSystem2664 : Subsystem
  Block8094 : Outport
  Block8095 : Outport  Port=2
  wires:
  Block8064/1 -> [TagName76]
  SubSystem2645/1(Output) -> Block8081/1
  SubSystem2646/1(Output) -> Block8081/2
  [TagName76] -> SubSystem2645/1(element), SubSystem2646/1(element)
  Block8081/1 -> Block8088/1
  SubSystem2664/1(Out1) -> Block8088/2
  Block8065/1 -> SubSystem2664/2(In2)  "mdl5_SubSystem2611_SubSystem2612_SubSystem2620_SubSystem2624_SubSystem2644_Block8065_1"
  Block8071/1 -> SubSystem2664/1(In1), SubSystem2659/1(In1), SubSystem2661/1(In1), SubSystem2660/1(In1), SubSystem2662/1(In1), SubSystem2663/1(In1)  "mdl5_SubSystem2611_SubSystem2612_SubSystem2620_SubSystem2624_SubSystem2644_Block8071_1"
  SubSystem2651/1(Output) -> Block8082/1
  SubSystem2652/1(Output) -> Block8082/2
  [TagName76] -> SubSystem2652/1(element), SubSystem2651/1(element)
  Block8082/1 -> Block8089/1
  SubSystem2653/1(Output) -> Block8083/1
  SubSystem2654/1(Output) -> Block8083/2
  [TagName76] -> SubSystem2653/1(element), SubSystem2654/1(element)
  Block8083/1 -> Block8090/1
  SubSystem2655/1(Output) -> Block8084/1
  SubSystem2656/1(Output) -> Block8084/2
  [TagName76] -> SubSystem2656/1(element), SubSystem2655/1(element)
  Block8084/1 -> Block8091/1
  SubSystem2657/1(Output) -> Block8085/1
  SubSystem2658/1(Output) -> Block8085/2
  [TagName76] -> SubSystem2657/1(element), SubSystem2658/1(element)
  Block8085/1 -> Block8092/1
  SubSystem2647/1(Output) -> Block8086/1
  SubSystem2648/1(Output) -> Block8086/2
  [TagName76] -> SubSystem2648/1(element), SubSystem2647/1(element)
  Block8086/1 -> Block8093/1
  SubSystem2649/1(Output) -> Block8087/1
  SubSystem2650/1(Output) -> Block8087/2
  [TagName76] -> SubSystem2649/1(element), SubSystem2650/1(element)
  Block8066/1 -> SubSystem2659/2(In2)  "mdl5_SubSystem2611_SubSystem2612_SubSystem2620_SubSystem2624_SubSystem2644_Block8066_1"
  Block8068/1 -> SubSystem2660/2(In2)  "mdl5_SubSystem2611_SubSystem2612_SubSystem2620_SubSystem2624_SubSystem2644_Block8068_1"
  Block8069/1 -> SubSystem2662/2(In2)  "mdl5_SubSystem2611_SubSystem2612_SubSystem2620_SubSystem2624_SubSystem2644_Block8069_1"
  SubSystem2659/1(Out1) -> Block8089/2
  SubSystem2661/1(Out1) -> Block8090/2
  SubSystem2660/1(Out1) -> Block8091/2
  SubSystem2662/1(Out1) -> Block8092/2
  SubSystem2663/1(Out1) -> Block8093/2
  Block8087/1 -> Block8093/3
  Block8089/1 -> Block8088/3  "mdl5_SubSystem2611_SubSystem2612_SubSystem2620_SubSystem2624_SubSystem2644_Block8089_1"
  Block8090/1 -> Block8089/3  "mdl5_SubSystem2611_SubSystem2612_SubSystem2620_SubSystem2624_SubSystem2644_Block8090_1"
  Block8091/1 -> Block8090/3  "mdl5_SubSystem2611_SubSystem2612_SubSystem2620_SubSystem2624_SubSystem2644_Block8091_1"
  Block8092/1 -> Block8091/3  "mdl5_SubSystem2611_SubSystem2612_SubSystem2620_SubSystem2624_SubSystem2644_Block8092_1"
  Block8093/1 -> Block8092/3  "mdl5_SubSystem2611_SubSystem2612_SubSystem2620_SubSystem2624_SubSystem2644_Block8093_1"
  Block8067/1 -> SubSystem2661/2(In2)  "mdl5_SubSystem2611_SubSystem2612_SubSystem2620_SubSystem2624_SubSystem2644_Block8067_1"
  Block8070/1 -> SubSystem2663/2(In2)  "mdl5_SubSystem2611_SubSystem2612_SubSystem2620_SubSystem2624_SubSystem2644_Block8070_1"
  Block8088/1 -> Block8072/1  "mdl5_SubSystem2611_SubSystem2612_SubSystem2620_SubSystem2624_SubSystem2644_Block8088_1"
  Block8072/1 -> Block8094/1
  Block8072/2 -> Block8095/1

== system mdl5/SubSystem2611/SubSystem2612/SubSystem2665/SubSystem2666/SubSystem2667 ==
  note: ***編集禁止***
  input : Inport
  element : Inport  Port=2
  Assignment : Assignment  IndexOptions=Index vector (port)  OutputSizes=[1 1]
  Inside_DSR : DataStoreRead  DataStoreName=DSM320
  Inside_DSW : DataStoreWrite  DataStoreName=DSM320
  wires:
  Assignment/1 -> Inside_DSW/1  "mdl5_SubSystem2611_SubSystem2612_SubSystem2665_SubSystem2666_SubSystem2667_Assignment_1"
  Inside_DSR/1 -> Assignment/1  "mdl5_SubSystem2611_SubSystem2612_SubSystem2665_SubSystem2666_SubSystem2667_Inside_DSR_1"
  input/1 -> Assignment/2
  element/1 -> Assignment/3

== system mdl5/SubSystem2611/SubSystem2612/SubSystem2665/SubSystem2666/SubSystem2668 ==
  note: ***編集禁止***
  In1 : Inport
  In2 : Inport  Port=2
  RO1 : RelationalOperator  Operator===  InputSameDT=on
  single1 : DataTypeConversion  OutDataTypeStr=single  SaturateOnIntegerOverflow=on  RndMeth=Zero
  single2 : DataTypeConversion  OutDataTypeStr=single  SaturateOnIntegerOverflow=on  RndMeth=Zero
  Out1 : Outport
  wires:
  RO1/1 -> Out1/1  "mdl5_SubSystem2611_SubSystem2612_SubSystem2665_SubSystem2666_SubSystem2668_RO1_1"
  In2/1 -> single2/1
  In1/1 -> single1/1
  single1/1 -> RO1/1  "mdl5_SubSystem2611_SubSystem2612_SubSystem2665_SubSystem2666_SubSystem2668_single1_1"
  single2/1 -> RO1/2  "mdl5_SubSystem2611_SubSystem2612_SubSystem2665_SubSystem2666_SubSystem2668_single2_1"

== system mdl5/SubSystem2611/SubSystem2612/SubSystem2665/SubSystem2666/SubSystem2669 ==
  note: ***編集禁止***
  In1 : Inport
  In2 : Inport  Port=2
  RO1 : RelationalOperator  Operator===  InputSameDT=on
  single1 : DataTypeConversion  OutDataTypeStr=single  SaturateOnIntegerOverflow=on  RndMeth=Zero
  single2 : DataTypeConversion  OutDataTypeStr=single  SaturateOnIntegerOverflow=on  RndMeth=Zero
  Out1 : Outport
  wires:
  RO1/1 -> Out1/1  "mdl5_SubSystem2611_SubSystem2612_SubSystem2665_SubSystem2666_SubSystem2669_RO1_1"
  In2/1 -> single2/1
  In1/1 -> single1/1
  single1/1 -> RO1/1  "mdl5_SubSystem2611_SubSystem2612_SubSystem2665_SubSystem2666_SubSystem2669_single1_1"
  single2/1 -> RO1/2  "mdl5_SubSystem2611_SubSystem2612_SubSystem2665_SubSystem2666_SubSystem2669_single2_1"

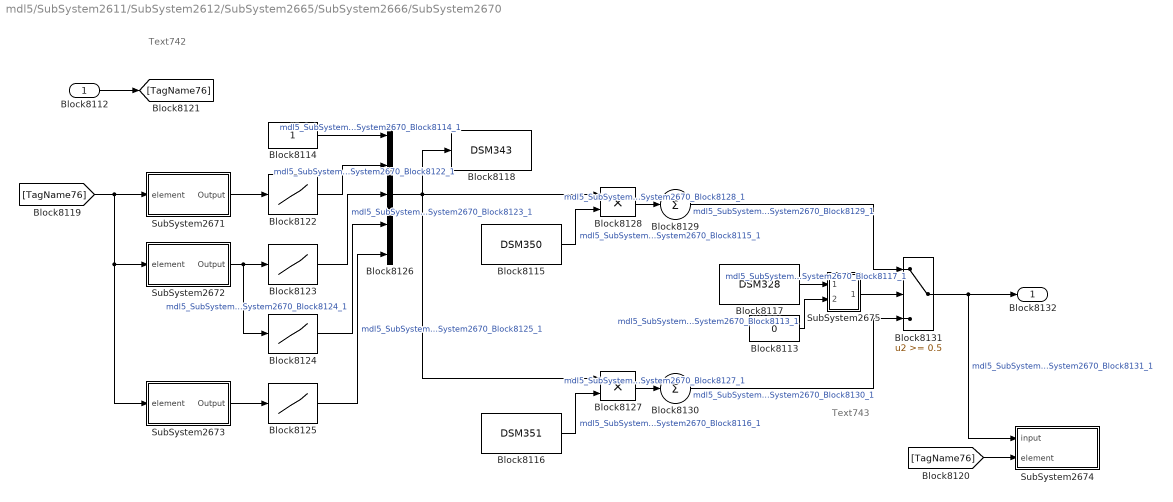
== system mdl5/SubSystem2611/SubSystem2612/SubSystem2665/SubSystem2666/SubSystem2670 ==
  note: Text743
  note: Text742
  Block8112 : Inport
  Block8113 : Constant  Value=0  OutDataTypeStr=double  SampleTime=-1
  Block8114 : Constant  OutDataTypeStr=double  SampleTime=-1
  Block8115 : DataStoreRead  DataStoreName=DSM350
  Block8116 : DataStoreRead  DataStoreName=DSM351
  Block8117 : DataStoreRead  DataStoreName=DSM328
  Block8118 : DataStoreWrite  DataStoreName=DSM343
  Block8122 : Lookup  InputValues=map_mr4_01  Table=map_mr4_02  SaturateOnIntegerOverflow=on
      settings: AttributesFormatString=<%<OutputValues>>\nAttribute2111
  Block8123 : Lookup  InputValues=map_mr4_03  Table=map_mr4_04  SaturateOnIntegerOverflow=on
      settings: AttributesFormatString=<%<OutputValues>>\nAttribute2112
  Block8124 : Lookup  InputValues=map_mr4_05  Table=map_mr4_06  SaturateOnIntegerOverflow=on
      settings: AttributesFormatString=<%<OutputValues>>\nAttribute2113
  Block8125 : Lookup  InputValues=map_mr4_07  Table=map_mr4_08  SaturateOnIntegerOverflow=on
      settings: AttributesFormatString=<%<OutputValues>>\nAttribute2114
  Block8126 : Mux  Inputs=5
  Block8127 : Product  OutDataTypeStr=double  SaturateOnIntegerOverflow=on  RndMeth=Zero  InputSameDT=on
  Block8128 : Product  OutDataTypeStr=double  SaturateOnIntegerOverflow=on  RndMeth=Zero  InputSameDT=on
  Block8129 : Sum  Inputs=+  OutDataTypeStr=double  RndMeth=Zero  SaturateOnIntegerOverflow=on  InputSameDT=on
  Block8130 : Sum  Inputs=+  OutDataTypeStr=double  RndMeth=Zero  SaturateOnIntegerOverflow=on  InputSameDT=on
  Block8131 : Switch  Threshold=0.5  RndMeth=Zero  SaturateOnIntegerOverflow=on  InputSameDT=on
  SubSystem2671 : Subsystem  TreatAsAtomicUnit=on  mask(***ATC.DSRVEC***){bd_version=1.01.A, r0=DSM97, r1=-1, r2=, r3=, r4=, r5=, r6=, r7=, r8=, r9=, c0=, c1=, c2=, c3=, c4=, c5=, c6=, c7=, c8=, c9=}
      mask prompts: bd_version "Version"
      mask help: これはAutoCからのブロックです．編集禁止．
      settings: OpenFcn=warndlg('変更禁止!');
      mask Help: web(ui_blockhelpmng(gcb));
      mask Display: disp('ATC.DSRVEC')
  SubSystem2672 : Subsystem  TreatAsAtomicUnit=on  mask(***ATC.DSRVEC***){bd_version=1.01.A, r0=DSM318, r1=-1, r2=, r3=, r4=, r5=, r6=, r7=, r8=, r9=, c0=, c1=, c2=, c3=, c4=, c5=, c6=, c7=, c8=, c9=}
      mask prompts: bd_version "Version"
      mask help: これはAutoCからのブロックです．編集禁止．
      settings: OpenFcn=warndlg('変更禁止!');
      mask Help: web(ui_blockhelpmng(gcb));
      mask Display: disp('ATC.DSRVEC')
  SubSystem2673 : Subsystem  TreatAsAtomicUnit=on  mask(***ATC.DSRVEC***){bd_version=1.01.A, r0=DSM36, r1=-1, r2=, r3=, r4=, r5=, r6=, r7=, r8=, r9=, c0=, c1=, c2=, c3=, c4=, c5=, c6=, c7=, c8=, c9=}
      mask prompts: bd_version "Version"
      mask help: これはAutoCからのブロックです．編集禁止．
      settings: OpenFcn=warndlg('変更禁止!');
      mask Help: web(ui_blockhelpmng(gcb));
      mask Display: disp('ATC.DSRVEC')
  SubSystem2674 : Subsystem  TreatAsAtomicUnit=on  mask(***ATC.DSWVEC***){bd_version=1.01.A, r0=DSM321, r1=-1, r2=, r3=, r4=, r5=, r6=, r7=, r8=, r9=, c0=, c1=, c2=, c3=, c4=, c5=, c6=, c7=, c8=, c9=}
      mask prompts: bd_version "Version"
      mask help: これはAutoCからのブロックです．編集禁止．
      settings: OpenFcn=warndlg('変更禁止!');
      mask Help: web(ui_blockhelpmng(gcb));
      mask Display: disp('ATC.DSRVEC')
  SubSystem2675 : Subsystem
  Block8132 : Outport
  wires:
  SubSystem2671/1(Output) -> Block8122/1
  SubSystem2672/1(Output) -> Block8124/1, Block8123/1
  SubSystem2673/1(Output) -> Block8125/1
  [TagName76] -> SubSystem2671/1(element), SubSystem2672/1(element), SubSystem2673/1(element)
  Block8126/1 -> Block8118/1, Block8128/1, Block8127/1
  Block8115/1 -> Block8128/2  "mdl5_SubSystem2611_SubSystem2612_SubSystem2665_SubSystem2666_SubSystem2670_Block8115_1"
  Block8116/1 -> Block8127/2  "mdl5_SubSystem2611_SubSystem2612_SubSystem2665_SubSystem2666_SubSystem2670_Block8116_1"
  Block8128/1 -> Block8129/1  "mdl5_SubSystem2611_SubSystem2612_SubSystem2665_SubSystem2666_SubSystem2670_Block8128_1"
  Block8131/1 -> Block8132/1, SubSystem2674/1(input)  "mdl5_SubSystem2611_SubSystem2612_SubSystem2665_SubSystem2666_SubSystem2670_Block8131_1"
  SubSystem2675/1(Out1) -> Block8131/2
  Block8117/1 -> SubSystem2675/1(In1)  "mdl5_SubSystem2611_SubSystem2612_SubSystem2665_SubSystem2666_SubSystem2670_Block8117_1"
  Block8113/1 -> SubSystem2675/2(In2)  "mdl5_SubSystem2611_SubSystem2612_SubSystem2665_SubSystem2666_SubSystem2670_Block8113_1"
  Block8127/1 -> Block8130/1  "mdl5_SubSystem2611_SubSystem2612_SubSystem2665_SubSystem2666_SubSystem2670_Block8127_1"
  Block8129/1 -> Block8131/1  "mdl5_SubSystem2611_SubSystem2612_SubSystem2665_SubSystem2666_SubSystem2670_Block8129_1"
  Block8114/1 -> Block8126/1  "mdl5_SubSystem2611_SubSystem2612_SubSystem2665_SubSystem2666_SubSystem2670_Block8114_1"
  Block8122/1 -> Block8126/2  "mdl5_SubSystem2611_SubSystem2612_SubSystem2665_SubSystem2666_SubSystem2670_Block8122_1"
  Block8123/1 -> Block8126/3  "mdl5_SubSystem2611_SubSystem2612_SubSystem2665_SubSystem2666_SubSystem2670_Block8123_1"
  Block8124/1 -> Block8126/4  "mdl5_SubSystem2611_SubSystem2612_SubSystem2665_SubSystem2666_SubSystem2670_Block8124_1"
  Block8125/1 -> Block8126/5  "mdl5_SubSystem2611_SubSystem2612_SubSystem2665_SubSystem2666_SubSystem2670_Block8125_1"
  [TagName76] -> SubSystem2674/2(element)
  Block8112/1 -> [TagName76]
  Block8130/1 -> Block8131/3  "mdl5_SubSystem2611_SubSystem2612_SubSystem2665_SubSystem2666_SubSystem2670_Block8130_1"
